simulink model "ESE4481ZController"  (R2024a)
settings: Solver=VariableStepAuto  StartTime=0.0  StopTime=10.0  RelTol=1e-3
undefined symbols (not defined in the file): Kpz, Kw, mass, Pdc
settings Model: Creator=achic  LastModifiedBy=achic

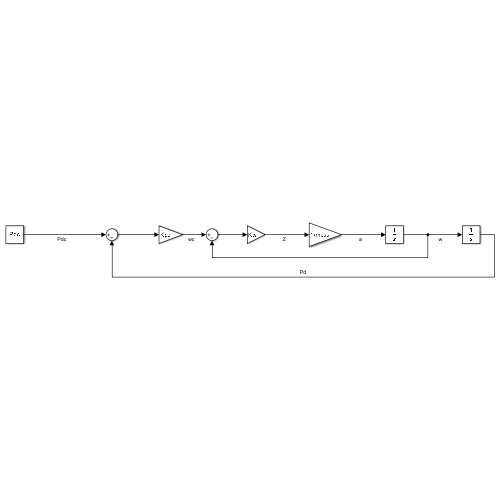
[thumbnail: Simulink's stored preview of the top-level diagram]
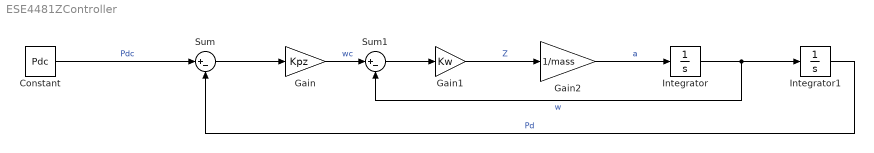
== system ESE4481ZController ==
  Constant : Constant  Value=Pdc
  Gain : Gain  Gain=Kpz
  Gain1 : Gain  Gain=Kw
  Gain2 : Gain  Gain=1/mass
  Integrator : Integrator
  Integrator1 : Integrator
  Sum : Sum  Inputs=|+-
  Sum1 : Sum  Inputs=|+-
  wires:
  Sum/1 -> Gain/1
  Gain/1 -> Sum1/1  "wc"
  Sum1/1 -> Gain1/1
  Gain2/1 -> Integrator/1  "a"
  Gain1/1 -> Gain2/1  "Z"
  Integrator/1 -> Sum1/2, Integrator1/1  "w"
  Integrator1/1 -> Sum/2  "Pd"
  Constant/1 -> Sum/1  "Pdc"
